simulink model "MatlabScheme"  (R2015b)
settings: Solver=VariableStepAuto  StartTime=0.0  StopTime=100  RelTol=1e-3
libraries: simulink x7
settings Model: Creator=zarar384  LastModifiedBy=zarar384

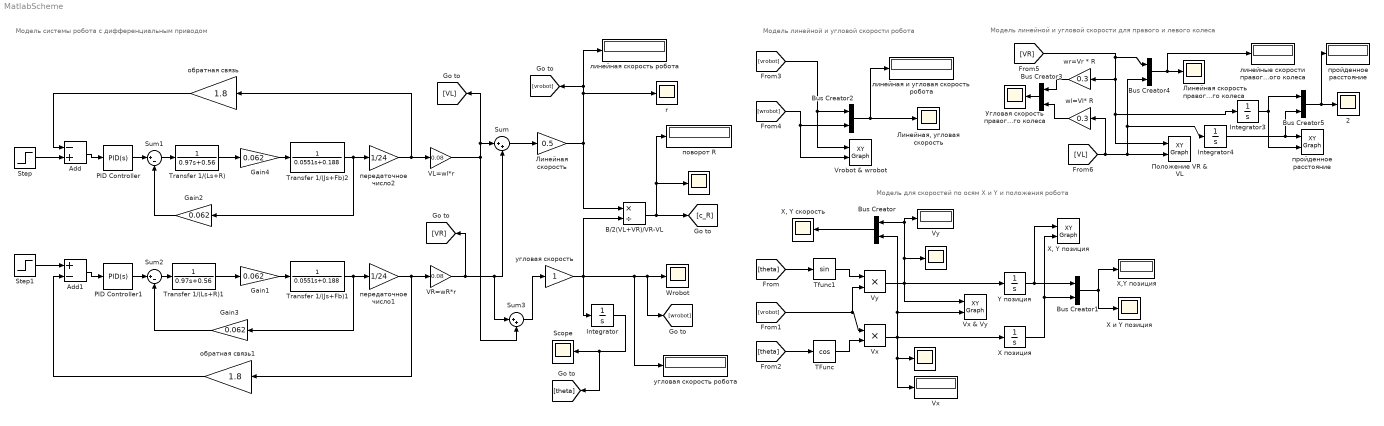
== system MatlabScheme ==
  note: Модель системы робота с дифференциальным приводом
  note: Модель линейной и угловой скорости для правого и левого колеса
  note: Модель линейной и угловой скорости робота
  note: Модель для скоростей по осям X и Y и положения робота
  " " : Scope
  "  " : Scope
  "   " : Scope
  "   X и Y позиция" : Scope
  "  2" : Scope
  Add : Sum  Inputs=-+
  Add1 : Sum  Inputs=+-
  B/2(VL+VR)/VR-VL : Product  Inputs=*/
  Bus Creator{,1..5} (6 alike) : BusCreator  Inputs=2
  Gain{1..4} (4 alike) : Gain  Gain=0.062
  Integrator : Integrator
  Integrator3 : Integrator
  Integrator4 : Integrator
  PID Controller : simulink/Continuous/PID Controller  Controller=PID  TimeDomain=Continuous-time  SampleTime=-1  IntegratorMethod=Forward Euler  FilterMethod=Forward Euler  Form=Parallel  UseFilter=on  ControllerParametersSource=internal  P=17.5  I=1.72  D=8  N=100  InitialConditionSource=internal  InitialConditionForIntegrator=0  InitialConditionForFilter=0  ExternalReset=none  LimitOutput=off  UpperSaturationLimit=inf  LowerSaturationLimit=-inf  LinearizeAsGain=on  AntiWindupMode=none  Kb=1  TrackingMode=off  Kt=1  PParamMin=[]  PParamMax=[]  IParamMin=[]  IParamMax=[]  DParamMin=[]  DParamMax=[]  NParamMin=[]  NParamMax=[]  KbParamMin=[]  KbParamMax=[]  KtParamMin=[]  KtParamMax=[]  POutMin=[]  POutMax=[]  IOutMin=[]  IOutMax=[]  DOutMin=[]  DOutMax=[]  NOutMin=[]  NOutMax=[]  KbOutMin=[]  KbOutMax=[]  KtOutMin=[]  KtOutMax=[]  IntegratorOutMin=[]  IntegratorOutMax=[]  FilterOutMin=[]  FilterOutMax=[]  SumOutMin=[]  SumOutMax=[]  SumI1OutMin=[]  SumI1OutMax=[]  SumI2OutMin=[]  SumI2OutMax=[]  SumI3OutMin=[]  SumI3OutMax=[]  SumDOutMin=[]  SumDOutMax=[]  SaturationOutMin=[]  SaturationOutMax=[]  IntegratorContinuousStateAttributes=''  IntegratorStateMustResolveToSignalObject=off  IntegratorRTWStateStorageClass=Auto  FilterContinuousStateAttributes=''  FilterStateMustResolveToSignalObject=off  FilterRTWStateStorageClass=Auto  DifferentiatorICPrevScaledInput=0  DifferentiatorOutMin=[]  DifferentiatorOutMax=[]
  PID Controller1 : simulink/Continuous/PID Controller  Controller=PID  TimeDomain=Continuous-time  SampleTime=-1  IntegratorMethod=Forward Euler  FilterMethod=Forward Euler  Form=Parallel  UseFilter=on  ControllerParametersSource=internal  P=17.5  I=1.72  D=8  N=100  InitialConditionSource=internal  InitialConditionForIntegrator=0  InitialConditionForFilter=0  ExternalReset=none  LimitOutput=off  UpperSaturationLimit=inf  LowerSaturationLimit=-inf  LinearizeAsGain=on  AntiWindupMode=none  Kb=1  TrackingMode=off  Kt=1  PParamMin=[]  PParamMax=[]  IParamMin=[]  IParamMax=[]  DParamMin=[]  DParamMax=[]  NParamMin=[]  NParamMax=[]  KbParamMin=[]  KbParamMax=[]  KtParamMin=[]  KtParamMax=[]  POutMin=[]  POutMax=[]  IOutMin=[]  IOutMax=[]  DOutMin=[]  DOutMax=[]  NOutMin=[]  NOutMax=[]  KbOutMin=[]  KbOutMax=[]  KtOutMin=[]  KtOutMax=[]  IntegratorOutMin=[]  IntegratorOutMax=[]  FilterOutMin=[]  FilterOutMax=[]  SumOutMin=[]  SumOutMax=[]  SumI1OutMin=[]  SumI1OutMax=[]  SumI2OutMin=[]  SumI2OutMax=[]  SumI3OutMin=[]  SumI3OutMax=[]  SumDOutMin=[]  SumDOutMax=[]  SaturationOutMin=[]  SaturationOutMax=[]  IntegratorContinuousStateAttributes=''  IntegratorStateMustResolveToSignalObject=off  IntegratorRTWStateStorageClass=Auto  FilterContinuousStateAttributes=''  FilterStateMustResolveToSignalObject=off  FilterRTWStateStorageClass=Auto  DifferentiatorICPrevScaledInput=0  DifferentiatorOutMin=[]  DifferentiatorOutMax=[]
  Scope : Scope
  Step : Step  After=12  SampleTime=0
  Step1 : Step  After=12  SampleTime=0
  Sum : Sum  Inputs=|++
  Sum1 : Sum  Inputs=|+-
  Sum2 : Sum  Inputs=|+-
  Sum3 : Sum  Inputs=|++
  TFunc : Trigonometry  Operator=cos
  Tfunc1 : Trigonometry
  Transfer 1/(Js+Fb)1 : TransferFcn  Denominator=[0.0551 0.188]
  Transfer 1/(Js+Fb)2 : TransferFcn  Denominator=[0.0551 0.188]
  Transfer 1/(Ls+R) : TransferFcn  Denominator=[0.97 0.56]
  Transfer 1/(Ls+R)1 : TransferFcn  Denominator=[0.97 0.56]
  VL=wl*r : Gain  Gain=0.08
  VR=wR*r : Gain  Gain=0.08
  Vrobot & wrobot : simulink/Sinks/XY Graph  xmin=-1  xmax=1  ymin=-1  ymax=1  st=-1
  Vx : Display
  "Vx " : Product
  Vx & Vy : simulink/Sinks/XY Graph  xmin=-0.5  xmax=0.5  ymin=-0.5  ymax=0.5  st=-1
  Vy : Display
  "Vy   " : Product
  Wrobot : Scope
  "X позиция " : Integrator
  "X, Y позиция" : simulink/Sinks/XY Graph  xmin=-1  xmax=1  ymin=-1  ymax=1  st=-1
  "X, Y скорость" : Scope
  X,Y позиция : Display
  Y позиция : Integrator
  r : Scope
  "wl=Vl* R " : Gain  Gain=0.3
  wr=Vr * R : Gain  Gain=0.3
  Линейная скорость : Gain  Gain=0.5
  Линейная скорость правого и левого колеса : Scope
  "Линейная, угловая скорость" : Scope
  Положение VR & VL : simulink/Sinks/XY Graph  xmin=-1  xmax=1  ymin=-1  ymax=1  st=-1
  "Угловая скорость правого и левого колеса " : Scope
  линейная и угловая скорость робота : Display
  "линейная скорость робота " : Display
  линейные скорости правого и левого колеса : Display
  обратная связь : Gain  Gain=1.8
  обратная связь1 : Gain  Gain=1.8
  передаточное число1 : Gain  Gain=1/24
  передаточное число2 : Gain  Gain=1/24
  поворот R : Display
  пройденное расстояние : simulink/Sinks/XY Graph  xmin=-1  xmax=1  ymin=-1  ymax=1  st=-1
  "пройденное расстояние\t" : Display
  угловая скорость : Gain
  угловая скорость робота : Display
  wires:
  Step/1 -> Add/2
  Add/1 -> PID Controller/1
  Transfer 1/(Ls+R)/1 -> Gain4/1
  Gain4/1 -> Transfer 1/(Js+Fb)2/1
  Transfer 1/(Js+Fb)2/1 -> Gain2/1, передаточное число2/1
  Gain2/1 -> Sum1/2
  PID Controller/1 -> Sum1/1
  Sum1/1 -> Transfer 1/(Ls+R)/1
  передаточное число2/1 -> обратная связь/1, VL=wl*r/1
  обратная связь/1 -> Add/1
  Add1/1 -> PID Controller1/1
  Transfer 1/(Ls+R)1/1 -> Gain1/1
  Transfer 1/(Js+Fb)1/1 -> передаточное число1/1, Gain3/1
  Gain3/1 -> Sum2/2
  PID Controller1/1 -> Sum2/1
  Sum2/1 -> Transfer 1/(Ls+R)1/1
  передаточное число1/1 -> обратная связь1/1, VR=wR*r/1
  Step1/1 -> Add1/1
  обратная связь1/1 -> Add1/2
  VR=wR*r/1 -> [VR], Sum3/1, Sum/2
  Sum/1 -> Линейная скорость/1
  Sum3/1 -> угловая скорость/1
  угловая скорость/1 -> угловая скорость робота/1, [wrobot], Wrobot/1, B/2(VL+VR)/VR-VL/2, Integrator/1
  Integrator/1 -> [theta], Scope/1
  B/2(VL+VR)/VR-VL/1 -> "   "/1, поворот R/1, [c_R]
  Линейная скорость/1 -> B/2(VL+VR)/VR-VL/1, [vrobot], "линейная скорость робота "/1, r/1
  Gain1/1 -> Transfer 1/(Js+Fb)1/1
  [theta] -> TFunc/1
  [theta] -> Tfunc1/1
  TFunc/1 -> "Vx "/2
  [vrobot] -> "Vy   "/2, "Vx "/1
  Tfunc1/1 -> "Vy   "/1
  "Vy   "/1 -> Vx & Vy/1, Vy/1, Bus Creator/1, " "/1, Y позиция/1
  "Vx "/1 -> "X позиция "/1, Vx/1, "  "/1, Vx & Vy/2, Bus Creator/2
  Y позиция/1 -> "X, Y позиция"/1, Bus Creator1/1
  "X позиция "/1 -> "X, Y позиция"/2, Bus Creator1/2
  Bus Creator1/1 -> "   X и Y позиция"/1, X,Y позиция/1
  Bus Creator/1 -> "X, Y скорость"/1
  Bus Creator2/1 -> линейная и угловая скорость робота/1, "Линейная, угловая скорость"/1
  [vrobot] -> Bus Creator2/1, Vrobot & wrobot/1
  [wrobot] -> Vrobot & wrobot/2, Bus Creator2/2
  wr=Vr * R/1 -> Bus Creator3/1
  "wl=Vl* R "/1 -> Bus Creator3/2
  Bus Creator3/1 -> "Угловая скорость правого и левого колеса "/1
  [VR] -> wr=Vr * R/1, Положение VR & VL/1, Integrator3/1, Bus Creator4/1
  [VL] -> "wl=Vl* R "/1, Bus Creator4/2, Integrator4/1, Положение VR & VL/2
  Bus Creator4/1 -> линейные скорости правого и левого колеса/1, Линейная скорость правого и левого колеса/1
  Integrator3/1 -> Bus Creator5/1, пройденное расстояние/2
  Integrator4/1 -> Bus Creator5/2, пройденное расстояние/1
  Bus Creator5/1 -> "пройденное расстояние\t"/1, "  2"/1
  VL=wl*r/1 -> Sum3/2, Sum/1, [VL]
